simulink model "doubleIT"  (R2018a)
settings: Solver=VariableStepAuto  StartTime=0.0  StopTime=10.0  RelTol=1e-3
libraries: simulink x1
settings Model: Creator=mattclark  LastModifiedBy=mattclark
settings SFSimCC: SimUserSources=doubleIT.c  SimUserLibraries=monitor.o
settings SFSimCC: SimCustomHeaderCode=|
  | #include "doubleIT.h"
  | #include "monitor.h"

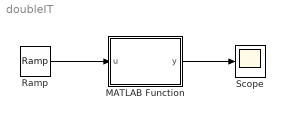
== system doubleIT ==
  MATLAB Function : MATLAB Function  TreatAsAtomicUnit=on
  Ramp : simulink/Sources/Ramp  slope=40  start=0  InitialOutput=-100
  Scope : Scope
  wires:
  Ramp/1 -> MATLAB Function/1(u)
  MATLAB Function/1(y) -> Scope/1

== matlab function doubleIT/MATLAB Function ==
  data: u input; y output
function y = doubleIT(u)
y = 0.0;
y = coder.ceval('doubleIT',u);
